simulink model "walkingstudy_nn_rigid_only"  (R2019a)
settings: Solver=FixedStepAuto  StartTime=0.0  StopTime=500  FixedStep=Ts  RelTol=1e-3  EnableMultiTasking=on
values from neighbouring files (symbols this model uses):
  f1_off = 0    [vreflex.m]
  f2_off = 0    [vreflex.m]
  f3_off = 0    [vreflex.m]
  f4_off = 0    [vreflex.m]
  f5_off = 0    [vreflex.m]
  f6_off = 0    [vreflex.m]
  trial = str2double(get(handles.tryno,'String'))    [vreflex.m]
  Ts = 0.0005    [vreflex.m]
  weight = evalin('base','weight')    [vreflex.m]
undefined symbols (not defined in the file or in its folder): DP_foot_gonio, filt_den, filt_num, foot_const, max_grf, max_phas, max_pos, min_grf, min_phas, min_pos, Pull, up
libraries: neural x30, dspsigops x17, speedgoatlib_IO183 x6, slrtlib x5, dspswit3 x1, dspstat3 x1
(part 1 of 2)
settings Model: Creator=vnalam  LastModifiedBy=vnalam
settings DataIOCC: LimitDataPoints=on  SaveFormat=StructureWithTime  ReturnWorkspaceOutputs=off
settings OptimizationCC: BlockReduction=off  OptimizeBlockIOStorage=off  BufferReuse=off  GlobalBufferReuse=off  ExpressionFolding=off  LocalBlockOutputs=off  LifeSpan=inf  OptimizeDataStoreBuffers=off  BusAssignmentInplaceUpdate=off
settings DebuggingCC: AllowSymbolicDim=off  SFUnexpectedBacktrackingDiag=warning  SFNoUnconditionalDefaultTransitionDiag=warning  SFExecutionAtInitializationDiag=none  ArithmeticOperatorsInVariantConditions=warning
settings HardwareCC: ProdBitPerPointer=32  ProdBitPerSizeT=32  ProdBitPerPtrDiffT=32  ProdLargestAtomicFloat=None  ProdWordSize=32  ProdLongLongMode=on  ProdHWDeviceType=Generic->32-bit x86 compatible
settings ModelReferenceCC: PropagateSignalLabelsOutOfModel=off
settings SFSimCC: SimUseLocalCustomCode=off
settings RTWCC: SystemTargetFile=slrt.tlc  TLCOptions=-axPCModelStackSizeKB=512  TemplateMakefile=slrt_default_tmf  Description=Simulink Real-Time  RTWUseLocalCustomCode=off  CodeExecutionProfiling=on  RTWCompilerOptimization=on
settings CodeAppCC: StateflowObjectComments=on
settings SimulinkRealTimeCC: PreserveStateflowLocalDataDimensions=off
settings ConfigComp: CovMetricSettings=dw  CovHtmlReporting=on  CovSaveCumulativeToWorkspaceVar=on  CovSaveSingleToWorkspaceVar=on  CovExternalEMLEnable=off

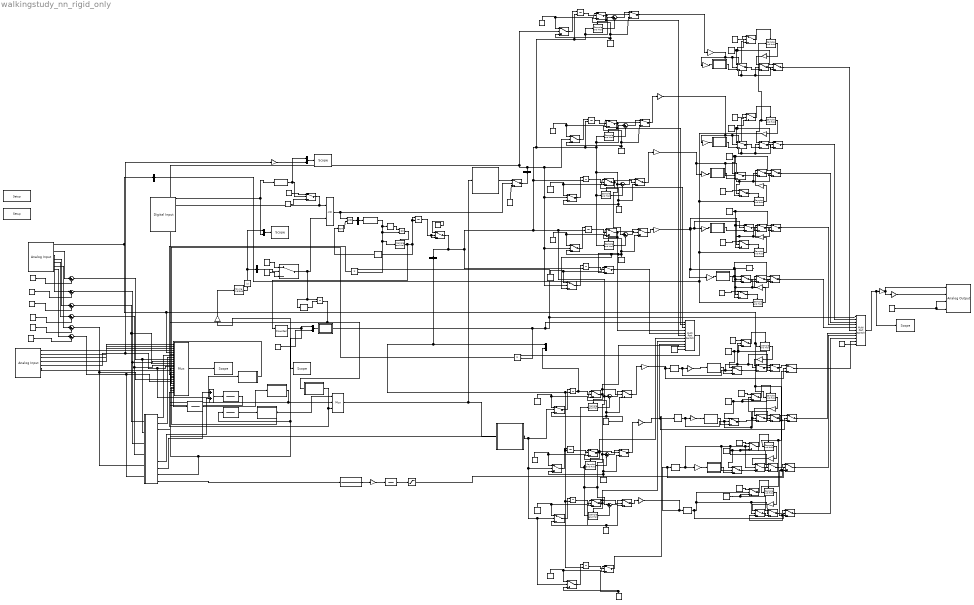
== system walkingstudy_nn_rigid_only ==
  note: RIGID
  Abs1 : Abs
  Add3 : Sum
  Analog Input : speedgoatlib_IO183/Analog Input  Priority=0  parModuleId=1  parSampTime=Ts  parPciSlot=-1  parAdChannelLow=1  parAdChannelHigh=8
      settings: SourceProductName=Simulink Real-Time: Speedgoat Library
  Analog Input1 : speedgoatlib_IO183/Analog Input  Priority=0  parModuleId=2  parSampTime=Ts  parPciSlot=-1  parAdChannelLow=1  parAdChannelHigh=8
      settings: SourceProductName=Simulink Real-Time: Speedgoat Library
  Analog Output : speedgoatlib_IO183/Analog Output  parModuleId=1  parSampTime=-1  parDaSimult=on  parPciSlot=-1  parDaChannels=[1 2 3 4]  parDaInit=[0 0 0 0]  parDaReset=[0 0 0 0]
      settings: SourceProductName=Simulink Real-Time: Speedgoat Library
  Constant{,3,7,10,12,14..16,18..19,27,29,31,35} (14 alike) : Constant  Value=0  SampleTime=Ts
  Constant{1,8,36,38,40,42,44,46,48} (9 alike) : Constant  SampleTime=-1
  Constant{9,11,34,37,39,41,43,45,47,49} (10 alike) : Constant  Value=0  SampleTime=-1
  Constant{2,4..6,13,17,26,28,30,32..33} (11 alike) : Constant  SampleTime=Ts
  Constant20 : Constant  Value=f1_off  SampleTime=Ts
  Constant21 : Constant  Value=f2_off  SampleTime=Ts
  Constant22 : Constant  Value=f3_off  SampleTime=Ts
  Constant23 : Constant  Value=f4_off  SampleTime=Ts
  Constant24 : Constant  Value=f6_off  SampleTime=Ts
  Constant25 : Constant  Value=f5_off  SampleTime=Ts
  Counter : dspswit3/Counter  Direction=Up  CountEvent=Rising edge  CounterSize=User defined  MaxCount=255  InitialCount=0  Output=Count and Hit  HitValue=32  ResetInput=on  SamplesPerFrame=1  Ts=1  CntDtype=double  HitDtype=Boolean
  Data Type Conversion1 : DataTypeConversion
  Data Type Conversion2 : DataTypeConversion
  Delay1 : Delay  DelayLength=12000  InitialCondition=0  SampleTime=Ts
  Delay{2..5} (4 alike) : Delay  DelayLength=60  InitialCondition=0  SampleTime=Ts
  Delay6 : Delay  DelayLength=1  InitialCondition=0  SampleTime=Ts
  Delay7 : Delay  DelayLength=1  InitialCondition=0  SampleTime=Ts
  Digital Input : speedgoatlib_IO183/Digital Input  parModuleId=2  parSampTime=-1  parPciSlot=-1  parDiChannels=[9 10 11 12 13 14 15 16]
      settings: SourceProductName=Simulink Real-Time: Speedgoat Library
  FIltered Fy : DiscreteFilter  Numerator=filt_num  Denominator=filt_den  InputProcessing=Columns as channels (frame based)  FilterStructure=Direct form II transposed  a0EqualsOne=on
  FIltered Pos : DiscreteFilter  Numerator=filt_num  Denominator=filt_den  InputProcessing=Columns as channels (frame based)  FilterStructure=Direct form II transposed  a0EqualsOne=on
  Filtered Weight : DiscreteFilter  Numerator=filt_num  Denominator=filt_den  InputProcessing=Columns as channels (frame based)  FilterStructure=Direct form II transposed  a0EqualsOne=on
  Function Fitting Neural Network : Subsystem
      mask help: Function Fitting Neural Network
      mask Display: e = 0.06;c1 = [120 150 230]/255;c2 = ([120 150 230]+0)/383;c3 = ([120 150 230]+128)/383;patch([0 1 1 0],[0 0 1 1],c1);patch([0 1 1 1-e 1-e 0+e],[0 0 1 1-e 0+e 0+e],c2);patch([0 0 1 1-e 0+e 0+e],[0 1 1 1-e 1-e 0+e],c3);plot([0 1 1 0 0],[0 0 1 1 0]);fprintf('NNET');port_label('input',1,' Input');port_label('output',1,'Output ');
  Function Fitting Neural Network1 : Subsystem
      mask help: Function Fitting Neural Network
      mask Display: e = 0.06;c1 = [120 150 230]/255;c2 = ([120 150 230]+0)/383;c3 = ([120 150 230]+128)/383;patch([0 1 1 0],[0 0 1 1],c1);patch([0 1 1 1-e 1-e 0+e],[0 0 1 1-e 0+e 0+e],c2);patch([0 0 1 1-e 0+e 0+e],[0 1 1 1-e 1-e 0+e],c3);plot([0 1 1 0 0],[0 0 1 1 0]);fprintf('NNET');port_label('input',1,' Input');port_label('output',1,'Output ');
  GRF Normalization1 : Subsystem
  Gain1 : Gain  Gain=-180/3.14
  Gain{2,12,14,32,34,37..38} (7 alike) : Gain  Gain=2000
  Gain{4,7,13,24..25,27,33,35} (8 alike) : Gain  Gain=1/250
  Gain{3,15,20..22,26,28,30..31} (9 alike) : Gain  Gain=-2
  Gain23 : Gain  Gain=1/40
  Gain36 : Gain  Gain=-1
  Gain5 : Gain  Gain=-1
  Gain6 : Gain  Gain=-1
  Healstrike Time Normalization 1 : Subsystem
  Integrator : Integrator  ExternalReset=rising
  Integrator{1..10} (10 alike) : Integrator  ExternalReset=falling
  Logical Operator : Logic  AllPortsSameDT=off  OutDataTypeStr=boolean
  Logical Operator2 : Logic  Operator=OR  AllPortsSameDT=off  OutDataTypeStr=boolean
  Logical Operator3 : Logic  Operator=NOT  AllPortsSameDT=off  OutDataTypeStr=boolean
  Logical Operator4 : Logic  AllPortsSameDT=off  OutDataTypeStr=boolean
  MATLAB Function : MATLAB Function  TreatAsAtomicUnit=on
  MATLAB Function1 : MATLAB Function  TreatAsAtomicUnit=on
  MATLAB Function2 : MATLAB Function  TreatAsAtomicUnit=on
  MATLAB Function3 : MATLAB Function  TreatAsAtomicUnit=on
  MATLAB Function4 : MATLAB Function  TreatAsAtomicUnit=on
  MATLAB Function5 : MATLAB Function  TreatAsAtomicUnit=on
  MATLAB Function6 : MATLAB Function  TreatAsAtomicUnit=on
  MATLAB Function7 : MATLAB Function  TreatAsAtomicUnit=on
  MATLAB Function8 : MATLAB Function  TreatAsAtomicUnit=on
  Moving Average : dspstat3/Moving Average  Method=Sliding window  ForgettingFactorPort=off  SpecifyWindowLength=on  WindowLength=4  ForgettingFactor=0.9  SimulateUsing=Code generation
  Multiport Switch1 : MultiPortSwitch  Inputs=10
  Multiport Switch4 : MultiPortSwitch  Inputs=10
  Mux{,1,5,8,13} (5 alike) : Mux  Inputs=1
  Mux{2..4,7} (4 alike) : Mux  Inputs=2
  Mux6 : Mux  Inputs=27
      settings: DisplayOption=signals
  Mux9 : Mux  Inputs=3
      settings: DisplayOption=signals
  Product13 : Product
  Product8 : Product
  "Raw Foot Normalization " : Subsystem
  Raw Foot Normalization 1 : Subsystem
  Sample and Hold{1..17} (17 alike) : dspsigops/Sample and Hold  trig=Rising edge  initCond=0  latchinput=off
  Saturation5 : Saturate  UpperLimit=100  LowerLimit=-100
  Scope 1 : slrtlib/Displays and Logging/Scope   scopeno=2  scopetype=Target  autostart=on  viewmode=Graphical sliding  formatstr='%15.6f'  grid=on  ylimits=[0,0]  nosamples=20000  noprepostsamples=0  interleave=1  triggermode=FreeRun  triggersignal=1  trigsignalfromport=off  triggerlevel=0.0  triggerslope=Either  triggerscope=1  triggersample=0  filename=tot303.dat  mode=Lazy  writesize=512  autorestart=off  dynamicfilemode=off  maxwritefilesize=512*1024^2
  Scope 2 : slrtlib/Displays and Logging/Scope   scopeno=1  scopetype=Target  autostart=on  viewmode=Numerical  formatstr='%15.6f'  grid=on  ylimits=[0,0]  nosamples=100  noprepostsamples=0  interleave=1  triggermode=FreeRun  triggersignal=1  trigsignalfromport=off  triggerlevel=0.0  triggerslope=Either  triggerscope=1  triggersample=0  filename=tot303.dat  mode=Lazy  writesize=512  autorestart=off  dynamicfilemode=off  maxwritefilesize=512*1024^2
  Scope 3 : slrtlib/Displays and Logging/Scope   scopeno=3  scopetype=File  autostart=on  viewmode=Graphical redraw  formatstr='%15.6f'  grid=on  ylimits=[0,0]  nosamples=1000000  noprepostsamples=0  interleave=1  triggermode=FreeRun  triggersignal=1  trigsignalfromport=off  triggerlevel=0.0  triggerslope=Either  triggerscope=1  triggersample=0  filename=OW01.dat  mode=Commit  writesize=1024  autorestart=off  dynamicfilemode=off  maxwritefilesize=512*1024^2
  Scope 4 : slrtlib/Displays and Logging/Scope   scopeno=4  scopetype=Target  autostart=on  viewmode=Graphical sliding  formatstr='%15.6f'  grid=on  ylimits=[0,0]  nosamples=20000  noprepostsamples=0  interleave=1  triggermode=FreeRun  triggersignal=1  trigsignalfromport=off  triggerlevel=0.0  triggerslope=Either  triggerscope=1  triggersample=0  filename=tot303.dat  mode=Lazy  writesize=512  autorestart=off  dynamicfilemode=off  maxwritefilesize=512*1024^2
  Scope 5 : slrtlib/Displays and Logging/Scope   scopeno=5  scopetype=Target  autostart=on  viewmode=Graphical sliding  formatstr='%15.6f'  grid=on  ylimits=[0,0]  nosamples=20000  noprepostsamples=0  interleave=1  triggermode=FreeRun  triggersignal=1  trigsignalfromport=off  triggerlevel=0.0  triggerslope=Either  triggerscope=1  triggersample=0  filename=tot303.dat  mode=Lazy  writesize=512  autorestart=off  dynamicfilemode=off  maxwritefilesize=512*1024^2
  Setup : speedgoatlib_IO183/Setup  parModuleId=1  parPciSlot=-1  parDaSimult=on  parAdCoupling=Single Ended  parAdRange=+-10V  parAdChannelLow=1  parAdChannelHigh=8  parDaChannels=[1:4]  parDaRange=0..5V  parDaInit=[0]  parDaReset=[0]  parDoChannels=[1:8]  parDoInit=[0]  parDoReset=[1]  parDiChannels=[9:16]  parIOPullReferenceFront=Pull-up (3.3V)  parIOPullReferenceRear=Pull-up (3.3V)
      settings: SourceProductName=Simulink Real-Time: Speedgoat Library
  Setup1 : speedgoatlib_IO183/Setup  parModuleId=2  parPciSlot=-1  parDaSimult=on  parAdCoupling=Single Ended  parAdRange=+-10V  parAdChannelLow=1  parAdChannelHigh=8  parDaChannels=[1:4]  parDaRange=0..5V  parDaInit=[0]  parDaReset=[0]  parDoChannels=[1:8]  parDoInit=[0]  parDoReset=[1]  parDiChannels=[9:16]  parIOPullReferenceFront=Pull-up (3.3V)  parIOPullReferenceRear=Pull-up (3.3V)
      settings: SourceProductName=Simulink Real-Time: Speedgoat Library
  Subsystem : Subsystem
  Sum{1..13} (13 alike) : Sum  Inputs=|+-
  Switch{1,7,12,16,64} (5 alike) : Switch  Criteria=u2 > Threshold  Threshold=4250
  Switch10 : Switch  Criteria=u2 > Threshold  Threshold=0.5
  Switch{11,20,25,33,41..42,44..45,47..48,50..51,53..54,56..58,60,62..63,68} (21 alike) : Switch  Criteria=u2 > Threshold
  Switch{4,8,13,17,67} (5 alike) : Switch  Criteria=u2 > Threshold  Threshold=5250
  Switch{2,9,14,18,65} (5 alike) : Switch  Criteria=u2 > Threshold  Threshold=4245
  Switch{15,34..39,66} (8 alike) : Switch  Criteria=u2 > Threshold  Threshold=250
  Switch{19,21,24,26} (4 alike) : Switch  Criteria=u2 > Threshold  Threshold=6245
  Switch{6,22,28,31} (4 alike) : Switch  Criteria=u2 > Threshold  Threshold=6250
  Switch{23,29..30,32} (4 alike) : Switch  Criteria=u2 > Threshold  Threshold=7250
  Switch27 : Switch  Criteria=u2 > Threshold  Threshold=1
  Switch3 : Switch  Criteria=u2 > Threshold  Threshold=31
  Switch40 : Switch  Criteria=u2 > Threshold  Threshold=5.9
  Switch43 : Switch  Criteria=u2 > Threshold  Threshold=44
  Switch46 : Switch  Criteria=u2 > Threshold  Threshold=57
  Switch49 : Switch  Criteria=u2 > Threshold  Threshold=16
  Switch5 : Switch  Criteria=u2 > Threshold  Threshold=weight*4/100
  Switch52 : Switch  Criteria=u2 > Threshold  Threshold=36
  Switch55 : Switch  Criteria=u2 > Threshold  Threshold=56
  Switch59 : Switch  Criteria=u2 > Threshold  Threshold=1
  Switch61 : Switch  Criteria=u2 > Threshold  Threshold=18
  Transfer Fcn1 : TransferFcn  Numerator=[1 0]  Denominator=[0.75 36.6606 700]
  Transfer Fcn3 : TransferFcn  Numerator=[30]  Denominator=[1 30]
  trial_V : Constant  Value=trial  SampleTime=Ts
  wires:
  Mux6/1 -> Scope 3/1
  Constant17/1 -> Switch5/1
  Constant18/1 -> Switch5/3
  Mux13/1 -> Switch5/2
  Data Type Conversion2/1 -> Mux3/1, Switch10/2
  Constant26/1 -> Switch10/1
  Sum1/1 -> Subsystem/2(In2), Mux6/9
  Sum2/1 -> Subsystem/3(In3), Mux6/10
  Sum3/1 -> Subsystem/1(In1), Mux6/11
  Sum6/1 -> Subsystem/4(In4), Mux6/12
  Sum8/1 -> Subsystem/6(In6), Mux6/21
  Analog Input1/2 -> Mux6/2
  Analog Input1/3 -> Mux6/3
  Analog Input1/1 -> Mux6/1
  Abs1/1 -> Mux4/1, Mux13/1
  Gain6/1 -> Moving Average/1
  Mux/1 -> Data Type Conversion1/1
  Delay1/1 -> Logical Operator2/1
  Logical Operator2/1 -> Sample and Hold1/Trigger
  Logical Operator/1 -> Mux/1
  Logical Operator3/1 -> Logical Operator/2
  Delay6/1 -> Logical Operator3/1
  Gain12/1 -> Gain24/1, Switch36/2, Switch4/2, Switch1/2, Switch2/2
  Data Type Conversion1/1 -> Product8/2, Sample and Hold1/1, Logical Operator2/2, Delay1/1
  Switch1/1 -> Switch4/3
  Gain14/1 -> Gain13/1, Switch35/2, Switch9/2, Switch8/2, Switch7/2
  Constant3/1 -> Switch35/1, Switch8/1, Switch9/3
  Switch7/1 -> Switch8/3
  Counter/1 -> Mux2/1, Scope 2/1
  MATLAB Function/1(y) -> Product13/2, Multiport Switch1/1, Product8/1, Multiport Switch4/1
  Product8/1 -> Mux6/17
  Gain23/1 -> Gain36/1, Analog Output/1
  Analog Input1/5 -> Gain5/1, Raw Foot Normalization 1/1(In1), Mux6/13
  Constant/1 -> Switch36/1, Switch2/3, Switch4/1
  Constant6/1 -> Switch2/1
  Switch2/1 -> Sample and Hold2/Trigger
  Sample and Hold2/1 -> Gain15/1
  Gain15/1 -> Switch1/1
  Switch9/1 -> Sample and Hold3/Trigger
  Constant2/1 -> Switch9/1
  Sample and Hold3/1 -> Gain20/1
  Gain20/1 -> Switch7/1
  Constant16/1 -> Analog Output/4, Analog Output/3
  Constant7/1 -> Switch34/1, Switch14/3, Switch13/1
  Switch12/1 -> Switch13/3
  Switch14/1 -> Sample and Hold4/Trigger
  Constant4/1 -> Switch14/1
  Sample and Hold4/1 -> Gain22/1
  Gain22/1 -> Switch12/1
  Gain25/1 -> MATLAB Function4/1(u)
  Constant10/1 -> Switch17/1, Switch18/3, Switch15/1
  Switch16/1 -> Switch17/3
  Switch15/1 -> Switch16/3
  Switch18/1 -> Sample and Hold5/Trigger
  Constant5/1 -> Switch18/1
  Sample and Hold5/1 -> Gain26/1
  Gain26/1 -> Switch16/1
  MATLAB Function4/1(y) -> Switch15/3
  Analog Input1/4 -> Mux6/4
  Constant27/1 -> Switch10/3
  Switch10/1 -> Logical Operator4/1, Mux6/6
  Analog Input/3 -> Sum1/1
  Analog Input/4 -> Sum2/1
  Analog Input/5 -> Sum3/1
  Analog Input/6 -> Sum6/1
  Constant20/1 -> Sum1/2
  Constant21/1 -> Sum2/2
  Constant22/1 -> Sum3/2
  Constant23/1 -> Sum6/2
  Analog Input/7 -> Sum7/1
  Constant25/1 -> Sum7/2
  Analog Input/8 -> Sum8/1
  Constant24/1 -> Sum8/2
  Logical Operator4/1 -> Switch68/2, Logical Operator/1
  Switch4/1 -> Multiport Switch4/2
  Switch8/1 -> Multiport Switch4/3
  Switch13/1 -> Multiport Switch4/4
  Switch17/1 -> Multiport Switch4/5
  Multiport Switch4/1 -> Scope 1/1, Gain23/1
  Gain1/1 -> Transfer Fcn3/1
  Transfer Fcn1/1 -> Gain1/1
  Transfer Fcn3/1 -> Saturation5/1
  Constant14/1 -> Switch37/1, Switch24/3, Switch30/1
  Switch6/1 -> Switch30/3
  Sample and Hold6/1 -> Gain21/1
  Switch31/1 -> Switch32/3
  Gain28/1 -> Switch31/1
  Constant32/1 -> Switch24/1
  Switch24/1 -> Sample and Hold6/Trigger
  Gain21/1 -> Switch6/1
  Constant28/1 -> Switch19/1
  Constant29/1 -> Switch38/1, Switch19/3, Switch32/1
  Switch19/1 -> Sample and Hold7/Trigger
  Sample and Hold7/1 -> Gain28/1
  Switch22/1 -> Switch23/3
  Gain31/1 -> Switch22/1
  Constant31/1 -> Switch39/1, Switch21/3, Switch23/1
  Switch21/1 -> Sample and Hold8/Trigger
  Sample and Hold8/1 -> Gain31/1
  Switch32/1 -> Switch11/1
  Switch30/1 -> Switch33/1
  Switch23/1 -> Switch20/1
  Constant30/1 -> Switch21/1
  Switch39/1 -> Switch22/3
  Saturation5/1 -> Switch28/3, Switch25/3, Switch33/3, Switch11/3, Switch20/3
  Gain32/1 -> Switch14/2, Switch13/2, Switch12/2, Switch34/2, Gain7/1, Gain25/1, Switch17/2, Switch16/2, Switch18/2, Switch15/2
  Switch28/1 -> Switch29/3
  Gain30/1 -> Switch28/1
  Constant15/1 -> Switch26/3, Switch29/1
  Switch26/1 -> Sample and Hold9/Trigger
  Sample and Hold9/1 -> Gain30/1
  Switch29/1 -> Switch25/1
  Constant33/1 -> Switch26/1
  Switch11/1 -> Multiport Switch4/7
  Switch20/1 -> Multiport Switch4/8
  Switch25/1 -> Multiport Switch4/9
  Mux2/1 -> MATLAB Function/1(u)
  trial_V/1 -> Mux2/2
  Gain7/1 -> MATLAB Function2/1(u)
  MATLAB Function2/1(y) -> Switch34/3
  Switch34/1 -> Switch12/3
  Gain13/1 -> MATLAB Function3/1(u)
  MATLAB Function3/1(y) -> Switch35/3
  Switch35/1 -> Switch7/3
  Gain24/1 -> MATLAB Function5/1(u)
  MATLAB Function5/1(y) -> Switch36/3
  Switch36/1 -> Switch1/3
  MATLAB Function6/1(y) -> Switch37/3
  Switch37/1 -> Switch6/3
  MATLAB Function7/1(y) -> Switch38/3
  Switch38/1 -> Switch31/3
  MATLAB Function8/1(y) -> Switch39/3
  Constant35/1 -> Switch40/1
  Sum7/1 -> Subsystem/5(In5), Mux6/20
  Gain36/1 -> Analog Output/2
  Analog Input1/6 -> Mux6/14
  Mux4/1 -> Scope 5/1
  Digital Input/1 -> Data Type Conversion2/1, Mux4/2
  Moving Average/1 -> Abs1/1
  Mux3/1 -> Scope 4/1
  Sample and Hold10/1 -> Sum4/2
  Sum4/1 -> Switch41/1
  Constant9/1 -> Switch42/3, Switch41/3, Switch3/3
  Constant8/1 -> Switch42/1, Switch3/1
  Switch3/1 -> Integrator1/1
  Integrator1/1 -> Switch42/2
  Switch42/1 -> Switch41/2, Sample and Hold10/Trigger, Multiport Switch1/2
  Constant36/1 -> Switch45/1, Switch43/1
  Constant37/1 -> Switch45/3, Switch44/3, Switch43/3
  Sample and Hold11/1 -> Sum5/2
  Integrator2/1 -> Switch45/2
  Switch45/1 -> Multiport Switch1/3, Sample and Hold11/Trigger, Switch44/2
  Sum5/1 -> Switch44/1
  Switch43/1 -> Integrator2/1
  Switch46/1 -> Integrator3/1
  Integrator3/1 -> Switch48/2
  Sample and Hold12/1 -> Sum9/2
  Sum9/1 -> Switch47/1
  Constant38/1 -> Switch48/1, Switch46/1
  Switch41/1 -> Gain12/1
  Switch44/1 -> Gain14/1
  Switch47/1 -> Gain32/1
  Constant44/1 -> Switch51/1, Switch49/1
  Switch56/1 -> Gain38/1
  Integrator4/1 -> Mux7/2, Switch51/2
  Switch50/1 -> Gain34/1
  Switch53/1 -> Gain37/1
  Sample and Hold1/1 -> Counter/1, Delay6/1, Integrator/1, Integrator/2
  Constant45/1 -> Switch51/3, Switch50/3, Switch49/3
  Sample and Hold13/1 -> Sum10/2
  Switch51/1 -> Multiport Switch1/10, Switch50/2, Sample and Hold13/Trigger
  Switch52/1 -> Integrator5/1
  Sum11/1 -> Switch53/1
  Switch54/1 -> Sample and Hold14/Trigger, Switch53/2, Multiport Switch1/7
  Gain37/1 -> Switch11/2, Delay3/1
  Constant41/1 -> Switch54/3, Switch53/3, Switch52/3
  Constant40/1 -> Switch54/1, Switch52/1
  Sample and Hold15/1 -> Sum12/2
  Constant43/1 -> Switch56/3, Switch57/3, Switch55/3
  Switch55/1 -> Integrator6/1
  Sum12/1 -> Switch56/1
  Switch57/1 -> Switch56/2, Multiport Switch1/8, Sample and Hold15/Trigger
  Integrator6/1 -> Switch57/2
  Integrator5/1 -> Switch54/2
  Sample and Hold14/1 -> Sum11/2
  Constant42/1 -> Switch57/1, Switch55/1
  Gain38/1 -> Delay5/1, Switch20/2, Delay4/1
  Sum10/1 -> Switch50/1
  Integrator/1 -> Switch40/3, Switch40/2
  Switch49/1 -> Integrator4/1
  Gain34/1 -> Switch33/2, Delay2/1
  Gain33/1 -> MATLAB Function7/1(u)
  Gain35/1 -> MATLAB Function8/1(u)
  Delay3/1 -> Switch19/2, Switch32/2, Switch31/2, Switch38/2, Gain33/1
  Delay4/1 -> Switch39/2, Switch23/2, Switch22/2, Switch21/2, Gain35/1
  Delay5/1 -> Switch25/2, Switch29/2, Switch28/2, Switch26/2
  Gain27/1 -> MATLAB Function6/1(u)
  Delay2/1 -> Switch30/2, Switch6/2, Switch24/2, Switch37/2, Gain27/1
  Multiport Switch1/1 -> Product13/1
  Product13/1 -> Mux6/22
  Mux9/1 -> Function Fitting Neural Network/1(Input), Function Fitting Neural Network1/1(Input)
  Switch5/1 -> Delay7/1, Integrator7/1, Logical Operator4/2
  Delay7/1 -> Integrator7/2
  Integrator7/1 -> Mux6/23, Healstrike Time Normalization 1/1(In1)
  Switch48/1 -> Sample and Hold12/Trigger, Multiport Switch1/4, Switch47/2
  Constant46/1 -> Switch58/1, Switch27/1
  Switch58/1 -> Multiport Switch1/9
  Integrator8/1 -> Switch58/2
  Switch27/1 -> Integrator8/1
  Constant47/1 -> Switch58/3, Switch27/3
  Function Fitting Neural Network1/1(Output) -> Switch27/2, Switch55/2, Switch52/2, Switch49/2, Mux6/16
  Mux8/1 -> Integrator8/2, Integrator6/2, Integrator5/2, Integrator4/2, Mux7/1
  Constant48/1 -> Switch60/1, Switch59/1
  Switch59/1 -> Integrator9/1
  Constant39/1 -> Switch48/3, Switch47/3, Switch60/3, Switch59/3, Switch46/3
  Integrator9/1 -> Switch60/2
  Switch60/1 -> Multiport Switch1/5
  Analog Input/1 -> Mux6/5, Sample and Hold6/1, Sample and Hold8/1, Sample and Hold9/1, Sample and Hold7/1, Mux1/1
  Subsystem/10(Out10) -> Gain6/1, Filtered Weight/1, Mux6/18
  Subsystem/1(Out1) -> Mux6/7
  Subsystem/2(Out2) -> Mux6/8
  Subsystem/3(Out3) -> Mux6/19
  Subsystem/8(Out8) -> Add3/2
  Subsystem/9(Out9) -> Add3/1
  Subsystem/11(Out11) -> Transfer Fcn1/1
  Switch63/1 -> Switch62/2, Multiport Switch1/6, Sample and Hold16/Trigger
  Sum13/1 -> Switch62/1
  Switch62/1 -> Gain2/1
  Integrator10/1 -> Switch63/2
  Switch61/1 -> Integrator10/1
  Sample and Hold16/1 -> Sum13/2
  Constant1/1 -> Switch63/1, Switch61/1
  Switch40/1 -> Integrator3/2, Sample and Hold13/1, Sample and Hold14/1, Sample and Hold15/1, Sum12/1, Sum11/1, Sum10/1, Integrator10/2, Sum13/1, Sample and Hold16/1, Integrator1/2, Sample and Hold12/1, Sample and Hold11/1, Sum9/1, Sum5/1, Sum4/1, Sample and Hold10/1, Integrator2/2, Integrator9/2, Mux8/1
  Constant11/1 -> Switch63/3, Switch62/3, Switch61/3
  Constant13/1 -> Switch65/1
  Mux1/1 -> Sample and Hold17/1, Sample and Hold2/1, Sample and Hold3/1, Sample and Hold4/1, Sample and Hold5/1
  Gain3/1 -> Switch64/1
  Gain2/1 -> Gain4/1, Switch66/2, Switch67/2, Switch64/2, Switch65/2
  Sample and Hold17/1 -> Gain3/1
  Switch66/1 -> Switch64/3
  Constant12/1 -> Switch66/1, Switch65/3, Switch67/1
  Switch64/1 -> Switch67/3
  Switch65/1 -> Sample and Hold17/Trigger
  Gain4/1 -> MATLAB Function1/1(u)
  MATLAB Function1/1(y) -> Switch66/3
  Switch67/1 -> Multiport Switch4/6
  Constant19/1 -> Multiport Switch4/11
  Constant34/1 -> Multiport Switch1/11
  Switch33/1 -> Multiport Switch4/10
  FIltered Fy/1 -> Mux6/25
  Filtered Weight/1 -> GRF Normalization1/1(In1)
  Add3/1 -> FIltered Fy/1
  "Raw Foot Normalization "/1(Out1) -> Mux9/2, Mux6/26
  Healstrike Time Normalization 1/1(Out1) -> Mux6/27, Mux9/3
  FIltered Pos/1 -> "Raw Foot Normalization "/1(In1)
  GRF Normalization1/1(Out1) -> Mux9/1, Mux6/24
  Raw Foot Normalization 1/1(Out1) -> FIltered Pos/1
  Constant49/1 -> Switch68/3
  Mux5/1 -> Mux6/15, Switch61/2, Switch3/2, Switch59/2, Switch46/2, Switch43/2
  Function Fitting Neural Network/1(Output) -> Switch68/1
  Switch68/1 -> Mux5/1
  Gain5/1 -> Mux3/2

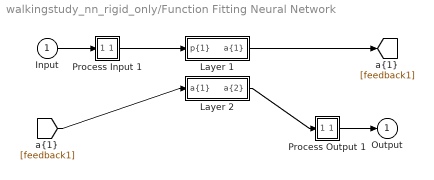
== system walkingstudy_nn_rigid_only/Function Fitting Neural Network ==
  Input : Inport  PortDimensions=3  SampleTime=0.0005
      mask Display: e = 0.06;c1 = [120 230 180]/255;c2 = ([120 230 180]+0)/(256+128);c3 = ([120 230 180]+128)/(256+128);patch([0 1 1 0],[0 0 1 1],c1);patch([0 1 1 1-e 1-e 0+e],[0 0 1 1-e 0+e 0+e],c2);patch([0 0 1 1-e 0+e 0+e],[0 1 1 1-e 1-e 0+e],c3);plot([0 1 1 0 0],[0 0 1 1 0]);
  Layer 1 : Subsystem
      mask Display: e = 0.06;c1 = [120 150 230]/255;c2 = ([120 150 230]+0)/383;c3 = ([120 150 230]+128)/383;patch([0 1 1 0],[0 0 1 1],c1);patch([0 1 1 1-e 1-e 0+e],[0 0 1 1-e 0+e 0+e],c2);patch([0 0 1 1-e 0+e 0+e],[0 1 1 1-e 1-e 0+e],c3);plot([0 1 1 0 0],[0 0 1 1 0]);
  Layer 2 : Subsystem
      mask Display: e = 0.06;c1 = [120 150 230]/255;c2 = ([120 150 230]+0)/383;c3 = ([120 150 230]+128)/383;patch([0 1 1 0],[0 0 1 1],c1);patch([0 1 1 1-e 1-e 0+e],[0 0 1 1-e 0+e 0+e],c2);patch([0 0 1 1-e 0+e 0+e],[0 1 1 1-e 1-e 0+e],c3);plot([0 1 1 0 0],[0 0 1 1 0]);
  Process Input 1 : Subsystem
      mask Display: e = 0.06;c1 = [120 150 230]/255;c2 = ([120 150 230]+0)/383;c3 = ([120 150 230]+128)/383;patch([0 1 1 0],[0 0 1 1],c1);patch([0 1 1 1-e 1-e 0+e],[0 0 1 1-e 0+e 0+e],c2);patch([0 0 1 1-e 0+e 0+e],[0 1 1 1-e 1-e 0+e],c3);plot([0 1 1 0 0],[0 0 1 1 0]);
  Process Output 1 : Subsystem
      mask Display: e = 0.06;c1 = [120 150 230]/255;c2 = ([120 150 230]+0)/383;c3 = ([120 150 230]+128)/383;patch([0 1 1 0],[0 0 1 1],c1);patch([0 1 1 1-e 1-e 0+e],[0 0 1 1-e 0+e 0+e],c2);patch([0 0 1 1-e 0+e 0+e],[0 1 1 1-e 1-e 0+e],c3);plot([0 1 1 0 0],[0 0 1 1 0]);
  Output : Outport  InitialOutput=0
      mask Display: e = 0.06;c1 = [120 230 180]/255;c2 = ([120 230 180]+0)/(256+128);c3 = ([120 230 180]+128)/(256+128);patch([0 1 1 0],[0 0 1 1],c1);patch([0 1 1 1-e 1-e 0+e],[0 0 1 1-e 0+e 0+e],c2);patch([0 0 1 1-e 0+e 0+e],[0 1 1 1-e 1-e 0+e],c3);plot([0 1 1 0 0],[0 0 1 1 0]);
  wires:
  Input/1 -> Process Input 1/1(x)
  Process Output 1/1(y) -> Output/1
  Process Input 1/1(p) -> Layer 1/1("p{1}")
  Layer 1/1("a{1}") -> [feedback1]
  [feedback1] -> Layer 2/1("a{1} ")
  Layer 2/1("a{2}") -> Process Output 1/1(a)

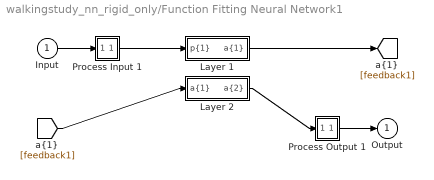
== system walkingstudy_nn_rigid_only/Function Fitting Neural Network1 ==
  Input : Inport  PortDimensions=3  SampleTime=0.0005
      mask Display: e = 0.06;c1 = [120 230 180]/255;c2 = ([120 230 180]+0)/(256+128);c3 = ([120 230 180]+128)/(256+128);patch([0 1 1 0],[0 0 1 1],c1);patch([0 1 1 1-e 1-e 0+e],[0 0 1 1-e 0+e 0+e],c2);patch([0 0 1 1-e 0+e 0+e],[0 1 1 1-e 1-e 0+e],c3);plot([0 1 1 0 0],[0 0 1 1 0]);
  Layer 1 : Subsystem
      mask Display: e = 0.06;c1 = [120 150 230]/255;c2 = ([120 150 230]+0)/383;c3 = ([120 150 230]+128)/383;patch([0 1 1 0],[0 0 1 1],c1);patch([0 1 1 1-e 1-e 0+e],[0 0 1 1-e 0+e 0+e],c2);patch([0 0 1 1-e 0+e 0+e],[0 1 1 1-e 1-e 0+e],c3);plot([0 1 1 0 0],[0 0 1 1 0]);
  Layer 2 : Subsystem
      mask Display: e = 0.06;c1 = [120 150 230]/255;c2 = ([120 150 230]+0)/383;c3 = ([120 150 230]+128)/383;patch([0 1 1 0],[0 0 1 1],c1);patch([0 1 1 1-e 1-e 0+e],[0 0 1 1-e 0+e 0+e],c2);patch([0 0 1 1-e 0+e 0+e],[0 1 1 1-e 1-e 0+e],c3);plot([0 1 1 0 0],[0 0 1 1 0]);
  Process Input 1 : Subsystem
      mask Display: e = 0.06;c1 = [120 150 230]/255;c2 = ([120 150 230]+0)/383;c3 = ([120 150 230]+128)/383;patch([0 1 1 0],[0 0 1 1],c1);patch([0 1 1 1-e 1-e 0+e],[0 0 1 1-e 0+e 0+e],c2);patch([0 0 1 1-e 0+e 0+e],[0 1 1 1-e 1-e 0+e],c3);plot([0 1 1 0 0],[0 0 1 1 0]);
  Process Output 1 : Subsystem
      mask Display: e = 0.06;c1 = [120 150 230]/255;c2 = ([120 150 230]+0)/383;c3 = ([120 150 230]+128)/383;patch([0 1 1 0],[0 0 1 1],c1);patch([0 1 1 1-e 1-e 0+e],[0 0 1 1-e 0+e 0+e],c2);patch([0 0 1 1-e 0+e 0+e],[0 1 1 1-e 1-e 0+e],c3);plot([0 1 1 0 0],[0 0 1 1 0]);
  Output : Outport  InitialOutput=0
      mask Display: e = 0.06;c1 = [120 230 180]/255;c2 = ([120 230 180]+0)/(256+128);c3 = ([120 230 180]+128)/(256+128);patch([0 1 1 0],[0 0 1 1],c1);patch([0 1 1 1-e 1-e 0+e],[0 0 1 1-e 0+e 0+e],c2);patch([0 0 1 1-e 0+e 0+e],[0 1 1 1-e 1-e 0+e],c3);plot([0 1 1 0 0],[0 0 1 1 0]);
  wires:
  Input/1 -> Process Input 1/1(x)
  Process Output 1/1(y) -> Output/1
  Process Input 1/1(p) -> Layer 1/1("p{1}")
  Layer 1/1("a{1}") -> [feedback1]
  [feedback1] -> Layer 2/1("a{1} ")
  Layer 2/1("a{2}") -> Process Output 1/1(a)

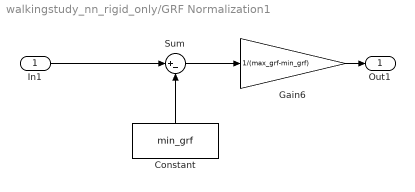
== system walkingstudy_nn_rigid_only/GRF Normalization1 ==
  In1 : Inport
  Constant : Constant  Value=min_grf
  Gain6 : Gain  Gain=1/(max_grf-min_grf)
  Sum : Sum  Inputs=|+-
  Out1 : Outport  VectorParamsAs1DForOutWhenUnconnected=on
  wires:
  In1/1 -> Sum/1
  Sum/1 -> Gain6/1
  Constant/1 -> Sum/2
  Gain6/1 -> Out1/1

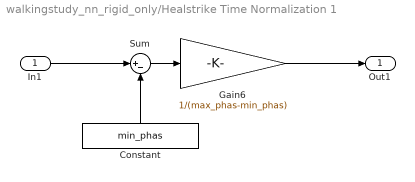
== system walkingstudy_nn_rigid_only/Healstrike Time Normalization 1 ==
  In1 : Inport
  Constant : Constant  Value=min_phas
  Gain6 : Gain  Gain=1/(max_phas-min_phas)
  Sum : Sum  Inputs=|+-
  Out1 : Outport  VectorParamsAs1DForOutWhenUnconnected=on
  wires:
  Gain6/1 -> Out1/1
  In1/1 -> Sum/1
  Sum/1 -> Gain6/1
  Constant/1 -> Sum/2

== system walkingstudy_nn_rigid_only/Raw Foot Normalization  ==
  In1 : Inport
  Constant : Constant  Value=min_pos
  Gain6 : Gain  Gain=1/(max_pos-min_pos)
  Sum : Sum  Inputs=|+-
  Out1 : Outport  VectorParamsAs1DForOutWhenUnconnected=on
  wires:
  Gain6/1 -> Out1/1
  Constant/1 -> Sum/2
  Sum/1 -> Gain6/1
  In1/1 -> Sum/1

== system walkingstudy_nn_rigid_only/Raw Foot Normalization 1 ==
  In1 : Inport
  Constant : Constant  Value=foot_const
  Gain6 : Gain  Gain=DP_foot_gonio*pi/180
  Sum : Sum  Inputs=|+-
  Out1 : Outport  VectorParamsAs1DForOutWhenUnconnected=on
  wires:
  Gain6/1 -> Out1/1
  Constant/1 -> Sum/2
  Sum/1 -> Gain6/1
  In1/1 -> Sum/1

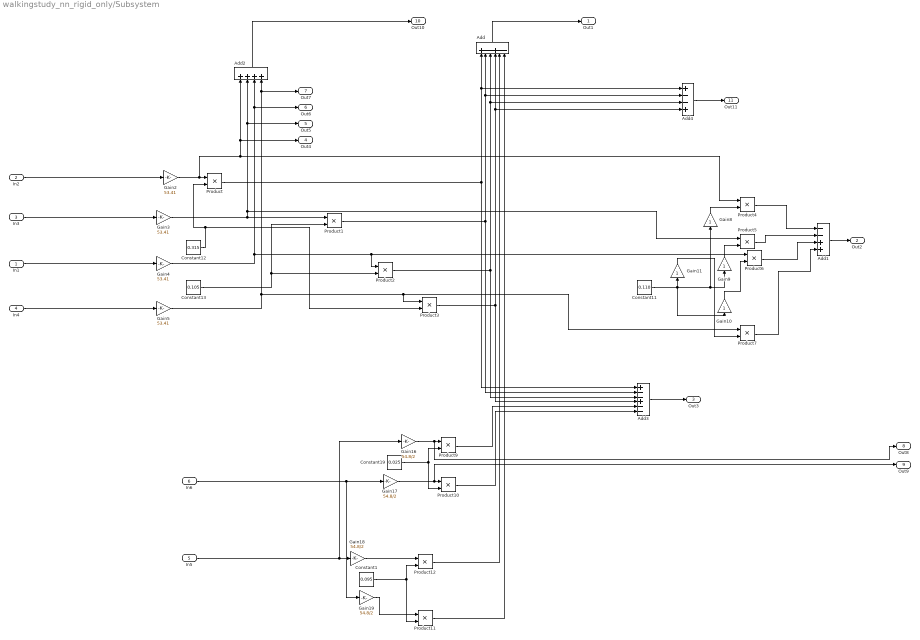
== system walkingstudy_nn_rigid_only/Subsystem ==
  In1 : Inport
  In2 : Inport  Port=2
  In3 : Inport  Port=3
  In4 : Inport  Port=4
  In5 : Inport  Port=5
  In6 : Inport  Port=6
  Add : Sum  Inputs=+--+--
  Add1 : Sum  Inputs=--++
  Add2 : Sum  Inputs=++++
  Add3 : Sum  Inputs=+--+--
  Add4 : Sum  Inputs=+--+
  Constant1 : Constant  Value=0.095  SampleTime=-1
  Constant11 : Constant  Value=0.110  SampleTime=-1
  Constant12 : Constant  Value=0.315  SampleTime=-1
  Constant13 : Constant  Value=0.105  SampleTime=-1
  Constant19 : Constant  Value=0.025  SampleTime=-1
  Gain{8..11} (4 alike) : Gain
  Gain{16..19} (4 alike) : Gain  Gain=54.8/2
  Gain{2..5} (4 alike) : Gain  Gain=53.41
  Product{,1..7,9..12} (12 alike) : Product
  Out1 : Outport  VectorParamsAs1DForOutWhenUnconnected=on
  Out2 : Outport  Port=2  VectorParamsAs1DForOutWhenUnconnected=on
  Out3 : Outport  Port=3  VectorParamsAs1DForOutWhenUnconnected=on
  Out4 : Outport  Port=4  VectorParamsAs1DForOutWhenUnconnected=on
  Out5 : Outport  Port=5  VectorParamsAs1DForOutWhenUnconnected=on
  Out6 : Outport  Port=6  VectorParamsAs1DForOutWhenUnconnected=on
  Out7 : Outport  Port=7  VectorParamsAs1DForOutWhenUnconnected=on
  Out8 : Outport  Port=8  VectorParamsAs1DForOutWhenUnconnected=on
  Out9 : Outport  Port=9  VectorParamsAs1DForOutWhenUnconnected=on
  Out10 : Outport  Port=10  VectorParamsAs1DForOutWhenUnconnected=on
  Out11 : Outport  Port=11  VectorParamsAs1DForOutWhenUnconnected=on
  wires:
  Gain4/1 -> Out6/1, Add2/3, Product6/1, Product2/1
  Gain3/1 -> Out5/1, Add2/2, Product5/1, Product1/1
  In3/1 -> Gain3/1
  Product2/1 -> Add3/3, Add4/3, Add/3
  Product1/1 -> Add4/2, Add/2, Add3/2
  Constant11/1 -> Gain11/1, Gain9/1, Gain8/1, Gain10/1
  Constant1/1 -> Product12/2, Product11/2
  Gain5/1 -> Product7/1, Product3/1, Add2/4, Out7/1
  In1/1 -> Gain4/1
  In6/1 -> Gain19/1, Gain17/1
  Product/1 -> Add4/1, Add/1, Add3/1
  Gain2/1 -> Product4/1, Add2/1, Out4/1, Product/1
  Product9/1 -> Add3/5
  In5/1 -> Gain16/1, Gain18/1
  Product10/1 -> Add3/6
  Gain19/1 -> Product11/1
  Product5/1 -> Add1/2
  In4/1 -> Gain5/1
  Constant12/1 -> Product/2, Product3/2
  Gain18/1 -> Product12/1
  Product6/1 -> Add1/3
  Product4/1 -> Add1/1
  Gain10/1 -> Product6/2
  Gain11/1 -> Product7/2
  Product12/1 -> Add/5
  Constant13/1 -> Product1/2, Product2/2
  Gain8/1 -> Product4/2
  Product3/1 -> Add/4, Add4/4, Add3/4
  Gain16/1 -> Out8/1, Product9/1
  Product7/1 -> Add1/4
  Gain9/1 -> Product5/2
  Product11/1 -> Add/6
  Add4/1 -> Out11/1
  Add2/1 -> Out10/1
  Gain17/1 -> Out9/1, Product10/1
  Constant19/1 -> Product9/2, Product10/2
  Add3/1 -> Out3/1
  In2/1 -> Gain2/1
  Add/1 -> Out1/1
  Add1/1 -> Out2/1

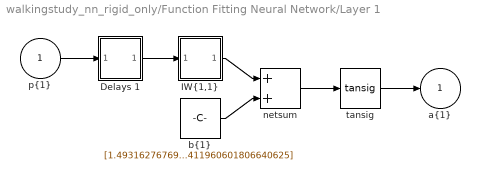
== system walkingstudy_nn_rigid_only/Function Fitting Neural Network/Layer 1 ==
  "p{1}" : Inport  PortDimensions=3  SampleTime=0.0005
      mask Display: e = 0.06;c1 = [120 230 180]/255;c2 = ([120 230 180]+0)/(256+128);c3 = ([120 230 180]+128)/(256+128);patch([0 1 1 0],[0 0 1 1],c1);patch([0 1 1 1-e 1-e 0+e],[0 0 1 1-e 0+e 0+e],c2);patch([0 0 1 1-e 0+e 0+e],[0 1 1 1-e 1-e 0+e],c3);plot([0 1 1 0 0],[0 0 1 1 0]);
  Delays 1 : Subsystem
      mask Display: e = 0.06;c1 = [120 150 230]/255;c2 = ([120 150 230]+0)/383;c3 = ([120 150 230]+128)/383;patch([0 1 1 0],[0 0 1 1],c1);patch([0 1 1 1-e 1-e 0+e],[0 0 1 1-e 0+e 0+e],c2);patch([0 0 1 1-e 0+e 0+e],[0 1 1 1-e 1-e 0+e],c3);plot([0 1 1 0 0],[0 0 1 1 0]);disp('0');
  "IW{1,1}" : Subsystem
      mask Display: e = 0.06;c1 = [120 150 230]/255;c2 = ([120 150 230]+0)/383;c3 = ([120 150 230]+128)/383;patch([0 1 1 0],[0 0 1 1],c1);patch([0 1 1 1-e 1-e 0+e],[0 0 1 1-e 0+e 0+e],c2);patch([0 0 1 1-e 0+e 0+e],[0 1 1 1-e 1-e 0+e],c3);plot([0 1 1 0 0],[0 0 1 1 0]);disp('W');
  "b{1}" : Constant  Value=[1.493162767693522408052331229555420577526092529296875;0.308878310747201123565019997840863652527332305908203125;2.418806707964403557298282976262271404266357421875;-0.53288467569516562161169304090435616672039031982421875;-1.9188256013522988485675568881561048328876495361328125;-0.359491402321449438073130977500113658607006072998046875;2.58424086724080925847601974965073168277740478515625;0.9172446137721923520302880206145346164703369140625;3.6865467233949242853441319311968982219696044921875;2.31201899257629239770039930590428411960601806640625]
      mask Display: e = 0.06;c1 = [120 150 230]/255;c2 = ([120 150 230]+0)/383;c3 = ([120 150 230]+128)/383;patch([0 1 1 0],[0 0 1 1],c1);patch([0 1 1 1-e 1-e 0+e],[0 0 1 1-e 0+e 0+e],c2);patch([0 0 1 1-e 0+e 0+e],[0 1 1 1-e 1-e 0+e],c3);plot([0 1 1 0 0],[0 0 1 1 0]);disp('b');
  netsum : Sum  Inputs=2  SaturateOnIntegerOverflow=on  InputSameDT=on  OutDataTypeStr=Inherit: Same as first input
      mask Display: e = 0.06;c1 = [120 150 230]/255;c2 = ([120 150 230]+0)/383;c3 = ([120 150 230]+128)/383;patch([0 1 1 0],[0 0 1 1],c1);patch([0 1 1 1-e 1-e 0+e],[0 0 1 1-e 0+e 0+e],c2);patch([0 0 1 1-e 0+e 0+e],[0 1 1 1-e 1-e 0+e],c3);plot([0 1 1 0 0],[0 0 1 1 0]);disp('+');
  tansig : neural/Transfer Functions/tansig
      settings: SourceProductName=MATLAB Runtime - Deep Learning Toolbox  SourceProductBaseCode=Missing
  "a{1}" : Outport  InitialOutput=[0;0;0;0;0;0;0;0;0;0]
      mask Display: e = 0.06;c1 = [120 230 180]/255;c2 = ([120 230 180]+0)/(256+128);c3 = ([120 230 180]+128)/(256+128);patch([0 1 1 0],[0 0 1 1],c1);patch([0 1 1 1-e 1-e 0+e],[0 0 1 1-e 0+e 0+e],c2);patch([0 0 1 1-e 0+e 0+e],[0 1 1 1-e 1-e 0+e],c3);plot([0 1 1 0 0],[0 0 1 1 0]);
  wires:
  "p{1}"/1 -> Delays 1/1("p{1}")
  Delays 1/1("pd{1,1}") -> "IW{1,1}"/1("pd{1,1}")
  "IW{1,1}"/1("iz{1,1}") -> netsum/1
  "b{1}"/1 -> netsum/2
  netsum/1 -> tansig/1
  tansig/1 -> "a{1}"/1

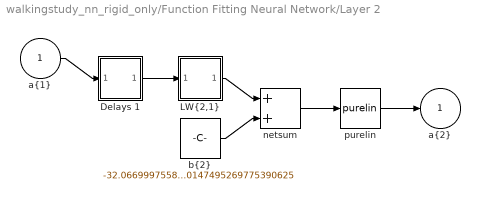
== system walkingstudy_nn_rigid_only/Function Fitting Neural Network/Layer 2 ==
  "a{1} " : Inport  PortDimensions=10  SampleTime=0.0005
      mask Display: e = 0.06;c1 = [120 230 180]/255;c2 = ([120 230 180]+0)/(256+128);c3 = ([120 230 180]+128)/(256+128);patch([0 1 1 0],[0 0 1 1],c1);patch([0 1 1 1-e 1-e 0+e],[0 0 1 1-e 0+e 0+e],c2);patch([0 0 1 1-e 0+e 0+e],[0 1 1 1-e 1-e 0+e],c3);plot([0 1 1 0 0],[0 0 1 1 0]);
  Delays 1 : Subsystem
      mask Display: e = 0.06;c1 = [120 150 230]/255;c2 = ([120 150 230]+0)/383;c3 = ([120 150 230]+128)/383;patch([0 1 1 0],[0 0 1 1],c1);patch([0 1 1 1-e 1-e 0+e],[0 0 1 1-e 0+e 0+e],c2);patch([0 0 1 1-e 0+e 0+e],[0 1 1 1-e 1-e 0+e],c3);plot([0 1 1 0 0],[0 0 1 1 0]);disp('0');
  "LW{2,1}" : Subsystem
      mask Display: e = 0.06;c1 = [120 150 230]/255;c2 = ([120 150 230]+0)/383;c3 = ([120 150 230]+128)/383;patch([0 1 1 0],[0 0 1 1],c1);patch([0 1 1 1-e 1-e 0+e],[0 0 1 1-e 0+e 0+e],c2);patch([0 0 1 1-e 0+e 0+e],[0 1 1 1-e 1-e 0+e],c3);plot([0 1 1 0 0],[0 0 1 1 0]);disp('W');
  "b{2}" : Constant  Value=-32.0669997558342316779089742340147495269775390625
      mask Display: e = 0.06;c1 = [120 150 230]/255;c2 = ([120 150 230]+0)/383;c3 = ([120 150 230]+128)/383;patch([0 1 1 0],[0 0 1 1],c1);patch([0 1 1 1-e 1-e 0+e],[0 0 1 1-e 0+e 0+e],c2);patch([0 0 1 1-e 0+e 0+e],[0 1 1 1-e 1-e 0+e],c3);plot([0 1 1 0 0],[0 0 1 1 0]);disp('b');
  netsum : Sum  Inputs=2  SaturateOnIntegerOverflow=on  InputSameDT=on  OutDataTypeStr=Inherit: Same as first input
      mask Display: e = 0.06;c1 = [120 150 230]/255;c2 = ([120 150 230]+0)/383;c3 = ([120 150 230]+128)/383;patch([0 1 1 0],[0 0 1 1],c1);patch([0 1 1 1-e 1-e 0+e],[0 0 1 1-e 0+e 0+e],c2);patch([0 0 1 1-e 0+e 0+e],[0 1 1 1-e 1-e 0+e],c3);plot([0 1 1 0 0],[0 0 1 1 0]);disp('+');
  purelin : neural/Transfer Functions/purelin
      settings: SourceProductName=MATLAB Runtime - Deep Learning Toolbox  SourceProductBaseCode=Missing
  "a{2}" : Outport  InitialOutput=0
      mask Display: e = 0.06;c1 = [120 230 180]/255;c2 = ([120 230 180]+0)/(256+128);c3 = ([120 230 180]+128)/(256+128);patch([0 1 1 0],[0 0 1 1],c1);patch([0 1 1 1-e 1-e 0+e],[0 0 1 1-e 0+e 0+e],c2);patch([0 0 1 1-e 0+e 0+e],[0 1 1 1-e 1-e 0+e],c3);plot([0 1 1 0 0],[0 0 1 1 0]);
  wires:
  "a{1} "/1 -> Delays 1/1("p{2}")
  Delays 1/1("pd{2,1}") -> "LW{2,1}"/1("ad{2,1}")
  "LW{2,1}"/1("lz{2,1}") -> netsum/1
  "b{2}"/1 -> netsum/2
  netsum/1 -> purelin/1
  purelin/1 -> "a{2}"/1

== system walkingstudy_nn_rigid_only/Function Fitting Neural Network/Process Input 1 ==
  x : Inport  PortDimensions=3  SampleTime=0.0005
      mask Display: e = 0.06;c1 = [120 230 180]/255;c2 = ([120 230 180]+0)/(256+128);c3 = ([120 230 180]+128)/(256+128);patch([0 1 1 0],[0 0 1 1],c1);patch([0 1 1 1-e 1-e 0+e],[0 0 1 1-e 0+e 0+e],c2);patch([0 0 1 1-e 0+e 0+e],[0 1 1 1-e 1-e 0+e],c3);plot([0 1 1 0 0],[0 0 1 1 0]);
  mapminmax : neural/Processing Functions/mapminmax  xmin=[0;0;0]  xmax=[1;1;1]  ymin=-1  ymax=1
      settings: SourceProductName=MATLAB Runtime - Deep Learning Toolbox  SourceProductBaseCode=Missing
  p : Outport  PortDimensions=3  SampleTime=0.0005
      mask Display: e = 0.06;c1 = [120 230 180]/255;c2 = ([120 230 180]+0)/(256+128);c3 = ([120 230 180]+128)/(256+128);patch([0 1 1 0],[0 0 1 1],c1);patch([0 1 1 1-e 1-e 0+e],[0 0 1 1-e 0+e 0+e],c2);patch([0 0 1 1-e 0+e 0+e],[0 1 1 1-e 1-e 0+e],c3);plot([0 1 1 0 0],[0 0 1 1 0]);
  wires:
  x/1 -> mapminmax/1
  mapminmax/1 -> p/1

== system walkingstudy_nn_rigid_only/Function Fitting Neural Network/Process Output 1 ==
  a : Inport  PortDimensions=1  SampleTime=0.0005
      mask Display: e = 0.06;c1 = [120 230 180]/255;c2 = ([120 230 180]+0)/(256+128);c3 = ([120 230 180]+128)/(256+128);patch([0 1 1 0],[0 0 1 1],c1);patch([0 1 1 1-e 1-e 0+e],[0 0 1 1-e 0+e 0+e],c2);patch([0 0 1 1-e 0+e 0+e],[0 1 1 1-e 1-e 0+e],c3);plot([0 1 1 0 0],[0 0 1 1 0]);
  mapminmax_reverse : neural/Processing Functions/mapminmax_reverse  xmin=0  xmax=100.000000000000014210854715202  ymin=-1  ymax=1
      settings: SourceProductName=MATLAB Runtime - Deep Learning Toolbox  SourceProductBaseCode=Missing
  y : Outport  PortDimensions=1  SampleTime=0.0005
      mask Display: e = 0.06;c1 = [120 230 180]/255;c2 = ([120 230 180]+0)/(256+128);c3 = ([120 230 180]+128)/(256+128);patch([0 1 1 0],[0 0 1 1],c1);patch([0 1 1 1-e 1-e 0+e],[0 0 1 1-e 0+e 0+e],c2);patch([0 0 1 1-e 0+e 0+e],[0 1 1 1-e 1-e 0+e],c3);plot([0 1 1 0 0],[0 0 1 1 0]);
  wires:
  a/1 -> mapminmax_reverse/1
  mapminmax_reverse/1 -> y/1

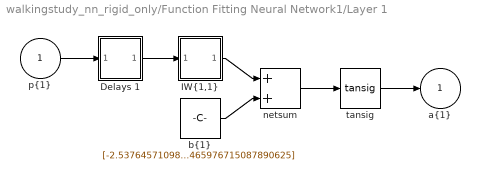
== system walkingstudy_nn_rigid_only/Function Fitting Neural Network1/Layer 1 ==
  "p{1}" : Inport  PortDimensions=3  SampleTime=0.0005
      mask Display: e = 0.06;c1 = [120 230 180]/255;c2 = ([120 230 180]+0)/(256+128);c3 = ([120 230 180]+128)/(256+128);patch([0 1 1 0],[0 0 1 1],c1);patch([0 1 1 1-e 1-e 0+e],[0 0 1 1-e 0+e 0+e],c2);patch([0 0 1 1-e 0+e 0+e],[0 1 1 1-e 1-e 0+e],c3);plot([0 1 1 0 0],[0 0 1 1 0]);
  Delays 1 : Subsystem
      mask Display: e = 0.06;c1 = [120 150 230]/255;c2 = ([120 150 230]+0)/383;c3 = ([120 150 230]+128)/383;patch([0 1 1 0],[0 0 1 1],c1);patch([0 1 1 1-e 1-e 0+e],[0 0 1 1-e 0+e 0+e],c2);patch([0 0 1 1-e 0+e 0+e],[0 1 1 1-e 1-e 0+e],c3);plot([0 1 1 0 0],[0 0 1 1 0]);disp('0');
  "IW{1,1}" : Subsystem
      mask Display: e = 0.06;c1 = [120 150 230]/255;c2 = ([120 150 230]+0)/383;c3 = ([120 150 230]+128)/383;patch([0 1 1 0],[0 0 1 1],c1);patch([0 1 1 1-e 1-e 0+e],[0 0 1 1-e 0+e 0+e],c2);patch([0 0 1 1-e 0+e 0+e],[0 1 1 1-e 1-e 0+e],c3);plot([0 1 1 0 0],[0 0 1 1 0]);disp('W');
  "b{1}" : Constant  Value=[-2.537645710986919933560557183227501809597015380859375;0.276037367021514878917543001080048270523548126220703125;-0.4096665771523946286691852947114966809749603271484375;0.436828686492216677894617760102846659719944000244140625;-0.439365501197540642142058686658856458961963653564453125;-1.9897585339451009378564094731700606644153594970703125;3.245988130280637040669944326509721577167510986328125;0.0004276456577187077198569375990899743555928580462932586669921875;-2.121871025031278445993621062370948493480682373046875;-2.26468871372382185569449575268663465976715087890625]
      mask Display: e = 0.06;c1 = [120 150 230]/255;c2 = ([120 150 230]+0)/383;c3 = ([120 150 230]+128)/383;patch([0 1 1 0],[0 0 1 1],c1);patch([0 1 1 1-e 1-e 0+e],[0 0 1 1-e 0+e 0+e],c2);patch([0 0 1 1-e 0+e 0+e],[0 1 1 1-e 1-e 0+e],c3);plot([0 1 1 0 0],[0 0 1 1 0]);disp('b');
  netsum : Sum  Inputs=2  SaturateOnIntegerOverflow=on  InputSameDT=on  OutDataTypeStr=Inherit: Same as first input
      mask Display: e = 0.06;c1 = [120 150 230]/255;c2 = ([120 150 230]+0)/383;c3 = ([120 150 230]+128)/383;patch([0 1 1 0],[0 0 1 1],c1);patch([0 1 1 1-e 1-e 0+e],[0 0 1 1-e 0+e 0+e],c2);patch([0 0 1 1-e 0+e 0+e],[0 1 1 1-e 1-e 0+e],c3);plot([0 1 1 0 0],[0 0 1 1 0]);disp('+');
  tansig : neural/Transfer Functions/tansig
      settings: SourceProductName=MATLAB Runtime - Deep Learning Toolbox  SourceProductBaseCode=Missing
  "a{1}" : Outport  InitialOutput=[0;0;0;0;0;0;0;0;0;0]
      mask Display: e = 0.06;c1 = [120 230 180]/255;c2 = ([120 230 180]+0)/(256+128);c3 = ([120 230 180]+128)/(256+128);patch([0 1 1 0],[0 0 1 1],c1);patch([0 1 1 1-e 1-e 0+e],[0 0 1 1-e 0+e 0+e],c2);patch([0 0 1 1-e 0+e 0+e],[0 1 1 1-e 1-e 0+e],c3);plot([0 1 1 0 0],[0 0 1 1 0]);
  wires:
  "p{1}"/1 -> Delays 1/1("p{1}")
  Delays 1/1("pd{1,1}") -> "IW{1,1}"/1("pd{1,1}")
  "IW{1,1}"/1("iz{1,1}") -> netsum/1
  "b{1}"/1 -> netsum/2
  netsum/1 -> tansig/1
  tansig/1 -> "a{1}"/1

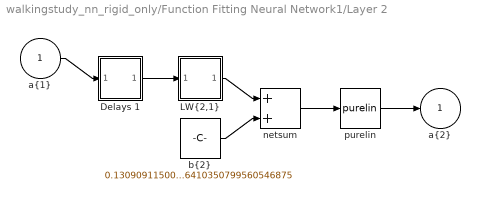
== system walkingstudy_nn_rigid_only/Function Fitting Neural Network1/Layer 2 ==
  "a{1} " : Inport  PortDimensions=10  SampleTime=0.0005
      mask Display: e = 0.06;c1 = [120 230 180]/255;c2 = ([120 230 180]+0)/(256+128);c3 = ([120 230 180]+128)/(256+128);patch([0 1 1 0],[0 0 1 1],c1);patch([0 1 1 1-e 1-e 0+e],[0 0 1 1-e 0+e 0+e],c2);patch([0 0 1 1-e 0+e 0+e],[0 1 1 1-e 1-e 0+e],c3);plot([0 1 1 0 0],[0 0 1 1 0]);
  Delays 1 : Subsystem
      mask Display: e = 0.06;c1 = [120 150 230]/255;c2 = ([120 150 230]+0)/383;c3 = ([120 150 230]+128)/383;patch([0 1 1 0],[0 0 1 1],c1);patch([0 1 1 1-e 1-e 0+e],[0 0 1 1-e 0+e 0+e],c2);patch([0 0 1 1-e 0+e 0+e],[0 1 1 1-e 1-e 0+e],c3);plot([0 1 1 0 0],[0 0 1 1 0]);disp('0');
  "LW{2,1}" : Subsystem
      mask Display: e = 0.06;c1 = [120 150 230]/255;c2 = ([120 150 230]+0)/383;c3 = ([120 150 230]+128)/383;patch([0 1 1 0],[0 0 1 1],c1);patch([0 1 1 1-e 1-e 0+e],[0 0 1 1-e 0+e 0+e],c2);patch([0 0 1 1-e 0+e 0+e],[0 1 1 1-e 1-e 0+e],c3);plot([0 1 1 0 0],[0 0 1 1 0]);disp('W');
  "b{2}" : Constant  Value=0.130909115008711107730476896904292516410350799560546875
      mask Display: e = 0.06;c1 = [120 150 230]/255;c2 = ([120 150 230]+0)/383;c3 = ([120 150 230]+128)/383;patch([0 1 1 0],[0 0 1 1],c1);patch([0 1 1 1-e 1-e 0+e],[0 0 1 1-e 0+e 0+e],c2);patch([0 0 1 1-e 0+e 0+e],[0 1 1 1-e 1-e 0+e],c3);plot([0 1 1 0 0],[0 0 1 1 0]);disp('b');
  netsum : Sum  Inputs=2  SaturateOnIntegerOverflow=on  InputSameDT=on  OutDataTypeStr=Inherit: Same as first input
      mask Display: e = 0.06;c1 = [120 150 230]/255;c2 = ([120 150 230]+0)/383;c3 = ([120 150 230]+128)/383;patch([0 1 1 0],[0 0 1 1],c1);patch([0 1 1 1-e 1-e 0+e],[0 0 1 1-e 0+e 0+e],c2);patch([0 0 1 1-e 0+e 0+e],[0 1 1 1-e 1-e 0+e],c3);plot([0 1 1 0 0],[0 0 1 1 0]);disp('+');
  purelin : neural/Transfer Functions/purelin
      settings: SourceProductName=MATLAB Runtime - Deep Learning Toolbox  SourceProductBaseCode=Missing
  "a{2}" : Outport  InitialOutput=0
      mask Display: e = 0.06;c1 = [120 230 180]/255;c2 = ([120 230 180]+0)/(256+128);c3 = ([120 230 180]+128)/(256+128);patch([0 1 1 0],[0 0 1 1],c1);patch([0 1 1 1-e 1-e 0+e],[0 0 1 1-e 0+e 0+e],c2);patch([0 0 1 1-e 0+e 0+e],[0 1 1 1-e 1-e 0+e],c3);plot([0 1 1 0 0],[0 0 1 1 0]);
  wires:
  "a{1} "/1 -> Delays 1/1("p{2}")
  Delays 1/1("pd{2,1}") -> "LW{2,1}"/1("ad{2,1}")
  "LW{2,1}"/1("lz{2,1}") -> netsum/1
  "b{2}"/1 -> netsum/2
  netsum/1 -> purelin/1
  purelin/1 -> "a{2}"/1

== system walkingstudy_nn_rigid_only/Function Fitting Neural Network1/Process Input 1 ==
  x : Inport  PortDimensions=3  SampleTime=0.0005
      mask Display: e = 0.06;c1 = [120 230 180]/255;c2 = ([120 230 180]+0)/(256+128);c3 = ([120 230 180]+128)/(256+128);patch([0 1 1 0],[0 0 1 1],c1);patch([0 1 1 1-e 1-e 0+e],[0 0 1 1-e 0+e 0+e],c2);patch([0 0 1 1-e 0+e 0+e],[0 1 1 1-e 1-e 0+e],c3);plot([0 1 1 0 0],[0 0 1 1 0]);
  mapminmax : neural/Processing Functions/mapminmax  xmin=[0;0.000170231830457990315590144358993;0]  xmax=[1;0.99426955886943202411742959157;1]  ymin=-1  ymax=1
      settings: SourceProductName=MATLAB Runtime - Deep Learning Toolbox  SourceProductBaseCode=Missing
  p : Outport  PortDimensions=3  SampleTime=0.0005
      mask Display: e = 0.06;c1 = [120 230 180]/255;c2 = ([120 230 180]+0)/(256+128);c3 = ([120 230 180]+128)/(256+128);patch([0 1 1 0],[0 0 1 1],c1);patch([0 1 1 1-e 1-e 0+e],[0 0 1 1-e 0+e 0+e],c2);patch([0 0 1 1-e 0+e 0+e],[0 1 1 1-e 1-e 0+e],c3);plot([0 1 1 0 0],[0 0 1 1 0]);
  wires:
  x/1 -> mapminmax/1
  mapminmax/1 -> p/1

== system walkingstudy_nn_rigid_only/Function Fitting Neural Network1/Process Output 1 ==
  a : Inport  PortDimensions=1  SampleTime=0.0005
      mask Display: e = 0.06;c1 = [120 230 180]/255;c2 = ([120 230 180]+0)/(256+128);c3 = ([120 230 180]+128)/(256+128);patch([0 1 1 0],[0 0 1 1],c1);patch([0 1 1 1-e 1-e 0+e],[0 0 1 1-e 0+e 0+e],c2);patch([0 0 1 1-e 0+e 0+e],[0 1 1 1-e 1-e 0+e],c3);plot([0 1 1 0 0],[0 0 1 1 0]);
  mapminmax_reverse : neural/Processing Functions/mapminmax_reverse  xmin=0  xmax=100.000000000000014210854715202  ymin=-1  ymax=1
      settings: SourceProductName=MATLAB Runtime - Deep Learning Toolbox  SourceProductBaseCode=Missing
  y : Outport  PortDimensions=1  SampleTime=0.0005
      mask Display: e = 0.06;c1 = [120 230 180]/255;c2 = ([120 230 180]+0)/(256+128);c3 = ([120 230 180]+128)/(256+128);patch([0 1 1 0],[0 0 1 1],c1);patch([0 1 1 1-e 1-e 0+e],[0 0 1 1-e 0+e 0+e],c2);patch([0 0 1 1-e 0+e 0+e],[0 1 1 1-e 1-e 0+e],c3);plot([0 1 1 0 0],[0 0 1 1 0]);
  wires:
  a/1 -> mapminmax_reverse/1
  mapminmax_reverse/1 -> y/1

== system walkingstudy_nn_rigid_only/Function Fitting Neural Network/Layer 1/Delays 1 ==
  "p{1}" : Inport  PortDimensions=3  SampleTime=0.0005
      mask Display: e = 0.06;c1 = [120 230 180]/255;c2 = ([120 230 180]+0)/(256+128);c3 = ([120 230 180]+128)/(256+128);patch([0 1 1 0],[0 0 1 1],c1);patch([0 1 1 1-e 1-e 0+e],[0 0 1 1-e 0+e 0+e],c2);patch([0 0 1 1-e 0+e 0+e],[0 1 1 1-e 1-e 0+e],c3);plot([0 1 1 0 0],[0 0 1 1 0]);
  mux : Mux  Inputs=1
      mask Display: e = 0.06;c1 = [120 150 230]/255;c2 = ([120 150 230]+0)/383;c3 = ([120 150 230]+128)/383;patch([0 1 1 0],[0 0 1 1],c1);patch([0 1 1 1-e 1-e 0+e],[0 0 1 1-e 0+e 0+e],c2);patch([0 0 1 1-e 0+e 0+e],[0 1 1 1-e 1-e 0+e],c3);plot([0 1 1 0 0],[0 0 1 1 0]);disp('Mux')
  "pd{1,1}" : Outport
      mask Display: e = 0.06;c1 = [120 230 180]/255;c2 = ([120 230 180]+0)/(256+128);c3 = ([120 230 180]+128)/(256+128);patch([0 1 1 0],[0 0 1 1],c1);patch([0 1 1 1-e 1-e 0+e],[0 0 1 1-e 0+e 0+e],c2);patch([0 0 1 1-e 0+e 0+e],[0 1 1 1-e 1-e 0+e],c3);plot([0 1 1 0 0],[0 0 1 1 0]);
  wires:
  "p{1}"/1 -> mux/1
  mux/1 -> "pd{1,1}"/1
